simulink model "thermal_closed_loop_model"  (R2023a)
settings: Solver=VariableStepAuto  StartTime=0.0  StopTime=600  RelTol=1e-3
PostLoadFcn:
  | run('thermal_plant_h2f175_parameters.m')
  | run('thermal_plant_peripherals_parameters.m')
  | run('thermal_variants_config.m')
undefined symbols (not defined in the file or in its folder): sigbuilder_block
libraries: simulink x1, nesl_utility x1
settings Model: Creator=adrian.taveras  LastModifiedBy=stefan.notter
settings OptimizationCC: ReuseModelBlockBuffer=off

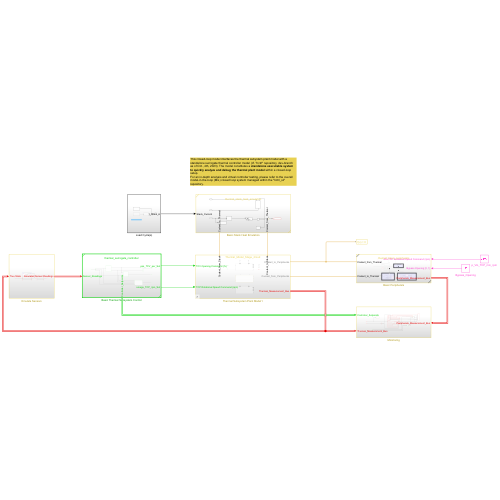
[thumbnail: Simulink's stored preview of the top-level diagram]
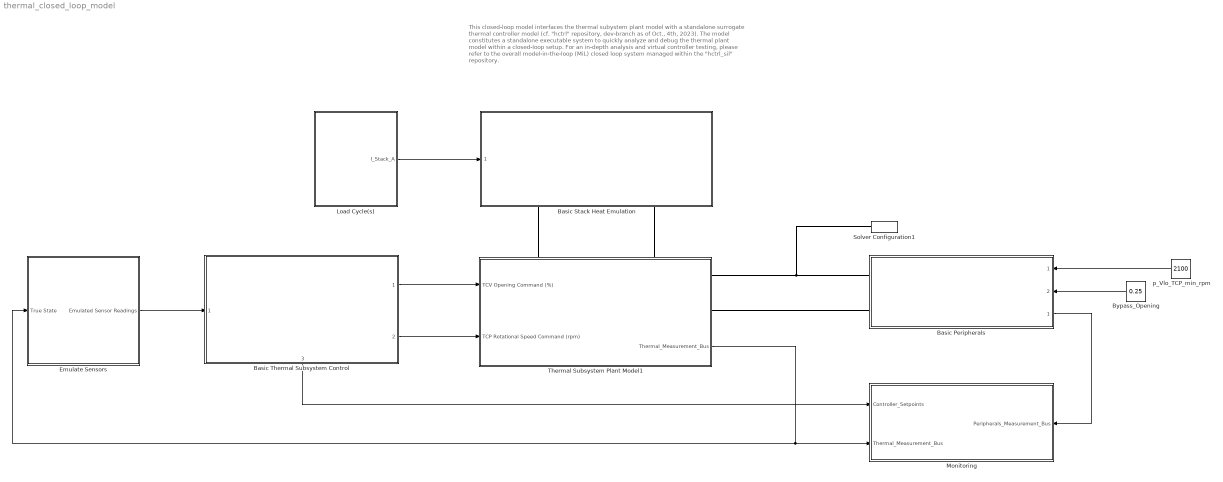
== system thermal_closed_loop_model ==
  note: This closed-loop model interfaces the thermal subystem plant model with a standalone surrogate thermal controller model (cf. "hctrl" repository, dev-branch as of Oct., 4th, 2023). The model constitutes a standalone executable system to quickly analyze and debug the thermal plant model within a closed-loop setup.
      | For an in-depth analysis and virtual controller testing, please refer to the overall model-in-the-loop (MiL) closed loop system managed within the "hctrl_sil" repository.
  Basic Peripherals : Subsystem  ReferencedSubsystem=thermal_basic_peripherals
      settings: PortSchema="{\"entries\":[{\"content\":{\"sides\":[{\"content\":{\"connectorIds\":[\"LConn1\",\"LConn2\"]},\"type\":\"ConnectorPlacement.EquallySpacedRectSide\",\"uuid\":\"3fb1bffc-06de-43a0-ba54-014616fc6cc1\"},{\"content\":{\"connectorIds\":[\"In1\",\"In2\",\"Out1\"],\"side\":\"RIGHT\"},\"type\":\"ConnectorPlacement.EquallySpacedRectSide\",\"uuid\":\"58405954-0a26-4c47-92cd-2c539f5c2dc2\"},{\"content\":{\"side\":\"TOP\"},\"type\":\"ConnectorPlacement.EquallySpacedRectSide\",\"uuid\":\"fb935e14-bdb8-42f8-ab88-5e819e25323e\"}]},\"type\":\"ConnectorPlacement.EquallySpacedConnector\",\"uuid\":\"bd863423-caf1-4028-a014-0e522635d1ca\"}],\"packageUris\":[\"http://schema.mathworks.com/mf0/Connector/R2020b\"],\"version\":\"1.0\"}"
  Basic Stack Heat Emulation : Subsystem  ReferencedSubsystem=thermal_stack_heat_emulation
      settings: PortSchema="{\"entries\":[{\"content\":{\"sides\":[{\"content\":{\"connectorIds\":[\"In1\"]},\"type\":\"ConnectorPlacement.EquallySpacedRectSide\",\"uuid\":\"3fb1bffc-06de-43a0-ba54-014616fc6cc1\"},{\"content\":{\"side\":\"RIGHT\"},\"type\":\"ConnectorPlacement.EquallySpacedRectSide\",\"uuid\":\"58405954-0a26-4c47-92cd-2c539f5c2dc2\"},{\"content\":{\"side\":\"TOP\"},\"type\":\"ConnectorPlacement.EquallySpacedRectSide\",\"uuid\":\"fb935e14-bdb8-42f8-ab88-5e819e25323e\"},{\"content\":{\"connectorIds\":[\"RConn1\",\"RConn2\"],\"side\":\"BOTTOM\"},\"type\":\"ConnectorPlacement.EquallySpacedRectSide\",\"uuid\":\"52bc4db1-df79-4132-9e52-2843fbef2d40\"}]},\"type\":\"ConnectorPlacement.EquallySpacedConnector\",\"uuid\":\"bd863423-caf1-4028-a014-0e522635d1ca\"}],\"packageUris\":[\"http://schema.mathworks.com/mf0/Connector/R2020b\"],\"version\":\"1.0\"}"
  Basic Thermal Subsystem Control : Subsystem  TreatAsAtomicUnit=on  SystemSampleTime=0.05  ReferencedSubsystem=thermal_surrogate_controller
      settings: RTWFcnNameOpts=Use subsystem name  RTWFileNameOpts=Use subsystem name  PortSchema="{\"entries\":[{\"content\":{\"sides\":[{\"content\":{\"connectorIds\":[\"In1\"]},\"type\":\"ConnectorPlacement.EquallySpacedRectSide\",\"uuid\":\"5ce399fd-075d-47cf-80d1-ee07a0b07c67\"},{\"content\":{\"connectorIds\":[\"Out1\",\"Out2\"],\"side\":\"RIGHT\"},\"type\":\"ConnectorPlacement.EquallySpacedRectSide\",\"uuid\":\"2f333d4b-83ed-4fad-b30d-41906106278f\"},{\"content\":{\"side\":\"TOP\"},\"type\":\"ConnectorPlacement.EquallySpacedRectSide\",\"uuid\":\"ce20a072-8b2c-48f8-86cd-e043d93c9dd9\"},{\"content\":{\"connectorIds\":[\"Out3\"],\"side\":\"BOTTOM\"},\"type\":\"ConnectorPlacement.EquallySpacedRectSide\",\"uuid\":\"72f45d63-3937-4d85-84da-630e4ae9e6af\"}]},\"type\":\"ConnectorPlacement.EquallySpacedConnector\",\"uuid\":\"e1990042-c5e7-41f2-bf10-f2665fc49181\"}],\"packageUris\":[\"http://schema.mathworks.com/mf0/Connector/R2020b\"],\"version\":\"1.0\"}"
  Bypass_Opening : Constant  Value=0.25
  Emulate Sensors : Subsystem
  Load Cycle(s) : Subsystem
  Monitoring : Subsystem
      settings: PortSchema="{\"entries\":[{\"content\":{\"sides\":[{\"content\":{\"connectorIds\":[\"In1\",\"In2\"]},\"type\":\"ConnectorPlacement.EquallySpacedRectSide\",\"uuid\":\"c7cb1208-b668-4b39-b890-dd3e20c5f08d\"},{\"content\":{\"connectorIds\":[\"In3\"],\"side\":\"RIGHT\"},\"type\":\"ConnectorPlacement.EquallySpacedRectSide\",\"uuid\":\"340204d2-358d-42ec-bbb6-f536bf598eab\"},{\"content\":{\"side\":\"TOP\"},\"type\":\"ConnectorPlacement.EquallySpacedRectSide\",\"uuid\":\"3db79fdc-6863-4ab5-88bc-fd1ec2b642bb\"}]},\"type\":\"ConnectorPlacement.EquallySpacedConnector\",\"uuid\":\"cd44049f-98c6-404f-bd6e-056e1be05d3b\"}],\"packageUris\":[\"http://schema.mathworks.com/mf0/Connector/R2020b\"],\"version\":\"1.0\"}"
  Solver Configuration1 : nesl_utility/Solver Configuration  PhysicalDomain=network_engine_domain  SubClassName=solver  LeftPortType=input  RightPortType=generic  Tones=[]  Harmonics=[]  SimulateNoise=off  Profile=off  UseLocalSampling=off  EnableSwitchedLinearOptims=on  FrequencyDomain=off  UseCCode=off  RelTol=0.001  AbsTol=1e-06  MinStep=1e-09  ToWorkspace=off  RevertToSquareIcSolve=off  NumHomotopyIterations=100  PhasorMode=off  PhasorModeNumHarmonics=1  ConsistencySolver=NEWTON_XTOL_AFTER_FTOL  IndexReductionMethod=DerivativeReplacement  DoDC=off  ResidualTolerance=1e-09  ConsistencyTolSource=GLOBAL  ConsistencyAbsTol=0.001  ConsistencyRelTol=0.001  ConsistencyTolFactor=0.001  UseLocalSolver=on  LocalSolverChoice=NE_BACKWARD_EULER_ADVANCER  ResolveIndetEquations=on  FunctionEvalNumThread=1  LocalSolverSampleTime=0.001  DoFixedCost=on  MaxNonlinIter=3  MaxModeIter=2  ComputeImpulses=off  ImpulseIterations=2  LinearAlgebra=auto  LinearAlgebraNumThread=0  EquationFormulation=NE_TIME_EF  DelaysMemoryBudget=1024  AutomaticFiltering=off  FilteringTimeConstant=0.001  PartitionStorageMethod=AS_NEEDED  PartitionMemoryBudget=1024  PartitionMethod=ROBUST
  Thermal Subsystem Plant Model1 : Subsystem  Variant=on
      settings: PortSchema="{\"entries\":[{\"content\":{\"sides\":[{\"content\":{\"connectorIds\":[\"In1\",\"In2\"]},\"type\":\"ConnectorPlacement.EquallySpacedRectSide\",\"uuid\":\"c406812b-8c92-4602-a172-62ad771a81a9\"},{\"content\":{\"connectorIds\":[\"RConn1\",\"RConn2\",\"Out1\"],\"side\":\"RIGHT\"},\"type\":\"ConnectorPlacement.EquallySpacedRectSide\",\"uuid\":\"78b6fff5-4256-4005-adaa-354cc2ed5b7d\"},{\"content\":{\"connectorIds\":[\"LConn1\",\"LConn2\"],\"side\":\"TOP\"},\"type\":\"ConnectorPlacement.EquallySpacedRectSide\",\"uuid\":\"1d5f4f72-4393-4f38-b9ce-f5bde53d6a3a\"}]},\"type\":\"ConnectorPlacement.EquallySpacedConnector\",\"uuid\":\"f62a8404-8485-4e42-883e-e8d18b630e2d\"}],\"packageUris\":[\"http://schema.mathworks.com/mf0/Connector/R2020b\"],\"version\":\"1.0\"}"
  p_Vlo_TCP_min_rpm : Constant  Value=2100
  wires:
  Emulate Sensors/1(Emulated Sensor Readings) -> Basic Thermal Subsystem Control/1
  p_Vlo_TCP_min_rpm/1 -> Basic Peripherals/1
  Load Cycle(s)/1(I_Stack_A) -> Basic Stack Heat Emulation/1
  Basic Peripherals/1 -> Monitoring/3(Peripherals_Measurement_Bus)
  Basic Thermal Subsystem Control/3 -> Monitoring/1(Controller_Setpoints)
  Bypass_Opening/1 -> Basic Peripherals/2
  Basic Thermal Subsystem Control/1 -> Thermal Subsystem Plant Model1/1(TCV Opening Command (%))
  Basic Thermal Subsystem Control/2 -> Thermal Subsystem Plant Model1/2(TCP Rotational Speed Command (rpm))
  Thermal Subsystem Plant Model1/1(Thermal_Measurement_Bus) -> Emulate Sensors/1(True State), Monitoring/2(Thermal_Measurement_Bus)
  connections:
  Thermal Subsystem Plant Model1/LConn2 -- Basic Stack Heat Emulation/RConn2
  Thermal Subsystem Plant Model1/LConn1 -- Basic Stack Heat Emulation/RConn1
  Thermal Subsystem Plant Model1/RConn1 -- Solver Configuration1/RConn1 -- Basic Peripherals/LConn1
  Thermal Subsystem Plant Model1/RConn2 -- Basic Peripherals/LConn2

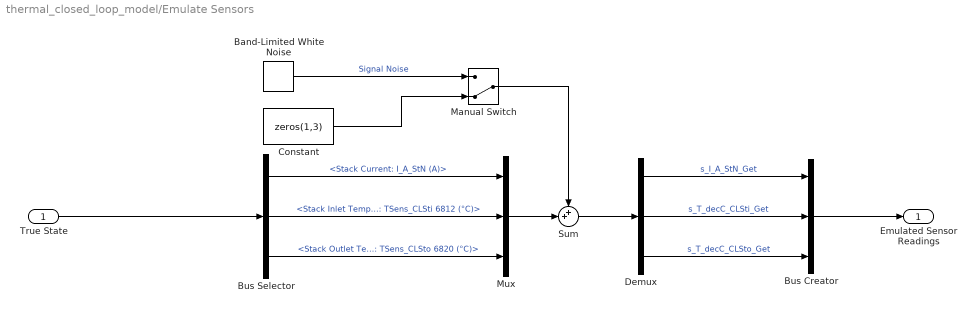
== system thermal_closed_loop_model/Emulate Sensors ==
  True State : Inport
  Band-Limited White Noise : simulink/Sources/Band-Limited White Noise  Cov=[5e-3, 5e-4, 5e-4]  Ts=0.1  seed=[23341]
  Bus Creator : BusCreator  Inputs=3
  Bus Selector : BusSelector  OutputSignals=Stack Current: I_A_StN (A),Stack Inlet Temperature: TSens_CLSti 6812 (°C),Stack Outlet Temperature: TSens_CLSto 6820 (°C)
  Constant : Constant  Value=zeros(1,3)
  Demux : Demux  Outputs=3
  Manual Switch : ManualSwitch  CurrentSetting=0
  Mux : Mux  Inputs=3
  Sum : Sum  Inputs=++|
  Emulated Sensor Readings : Outport
  wires:
  Bus Creator/1 -> Emulated Sensor Readings/1
  True State/1 -> Bus Selector/1
  Bus Selector/1 -> Mux/1  "<Stack Current: I_A_StN (A)>"
  Bus Selector/2 -> Mux/2  "<Stack Inlet Temperature: TSens_CLSti 6812 (°C)>"
  Bus Selector/3 -> Mux/3  "<Stack Outlet Temperature: TSens_CLSto 6820 (°C)>"
  Mux/1 -> Sum/2
  Sum/1 -> Demux/1
  Manual Switch/1 -> Sum/1
  Band-Limited White Noise/1 -> Manual Switch/1  "Signal Noise"
  Constant/1 -> Manual Switch/2
  Demux/1 -> Bus Creator/1  "s_I_A_StN_Get"
  Demux/3 -> Bus Creator/3  "s_T_decC_CLSto_Get"
  Demux/2 -> Bus Creator/2  "s_T_decC_CLSti_Get"

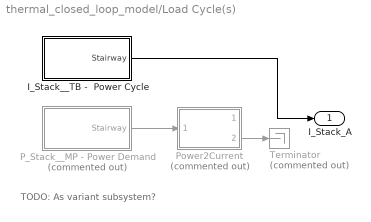
== system thermal_closed_loop_model/Load Cycle(s) ==
  note: TODO: As variant subsystem?
  I_Stack__TB -  Power Cycle : Subsystem  Tag=STV Subsys  LoadFcn=sigbuilder_block('load');  StartFcn=sigbuilder_block('start');  StopFcn=sigbuilder_block('stop');  ClipboardFcn=sigbuilder_block('clipboard');  mask(Sigbuilder block){tuvar=[0:10]}
      mask help: Simulink:masks:SigbuilderBlock_MD
      mask init:
      | if ~strcmp(get_param(bdroot(gcbh),'SimulationStatus'),'stopped') tuvar = sigbuilder_block('maskInit'); end
      settings: CopyFcn=sigbuilder_block('copy');  DeleteFcn=sigbuilder_block('delete');  ModelCloseFcn=sigbuilder_block('modelClose');  PreSaveFcn=sigbuilder_block('preSave');  PauseFcn=sigbuilder_block('pause');  ContinueFcn=sigbuilder_block('continue');  NameChangeFcn=sigbuilder_block('namechange');  OpenFcn=sigbuilder_block('open',[150.6 139.8 551.4 322.2 ]);  CloseFcn=sigbuilder_block('close');
      mask Display: plot(0, 0, 100, 100,[2, 2, 32, 32, 2], [68, 8, 8, 68, 68],[32, 2], [38, 38], [32, 19, 2],[53, 60, 44], [32, 17, 17, 2],[16, 16, 31, 31]);txt = getActiveGroup(gcbh);text(2, 100, txt,'verticalAlignment', 'top');
  P_Stack__MP - Power Demand : Subsystem  Tag=STV Subsys  Commented=on  LoadFcn=sigbuilder_block('load');  StartFcn=sigbuilder_block('start');  StopFcn=sigbuilder_block('stop');  ClipboardFcn=sigbuilder_block('clipboard');  mask(Sigbuilder block){tuvar=[0:10]}
      mask help: Simulink:masks:SigbuilderBlock_MD
      mask init:
      | if ~strcmp(get_param(bdroot(gcbh),'SimulationStatus'),'stopped') tuvar = sigbuilder_block('maskInit'); end
      settings: CopyFcn=sigbuilder_block('copy');  DeleteFcn=sigbuilder_block('delete');  ModelCloseFcn=sigbuilder_block('modelClose');  PreSaveFcn=sigbuilder_block('preSave');  PauseFcn=sigbuilder_block('pause');  ContinueFcn=sigbuilder_block('continue');  NameChangeFcn=sigbuilder_block('namechange');  OpenFcn=sigbuilder_block('open',[5.4 5.4 1141.2 580.8 ]);  CloseFcn=sigbuilder_block('close');
      mask Display: plot(0, 0, 100, 100,[2, 2, 32, 32, 2], [68, 8, 8, 68, 68],[32, 2], [38, 38], [32, 19, 2],[53, 60, 44], [32, 17, 17, 2],[16, 16, 31, 31]);txt = getActiveGroup(gcbh);text(2, 100, txt,'verticalAlignment', 'top');
  Power2Current : Subsystem  Commented=on
  Terminator : Terminator  Commented=on
  I_Stack_A : Outport
  wires:
  P_Stack__MP - Power Demand/1(Stairway) -> Power2Current/1(P_Stack)
  Power2Current/2(V_Stack) -> Terminator/1
  I_Stack__TB -  Power Cycle/1(Stairway) -> I_Stack_A/1

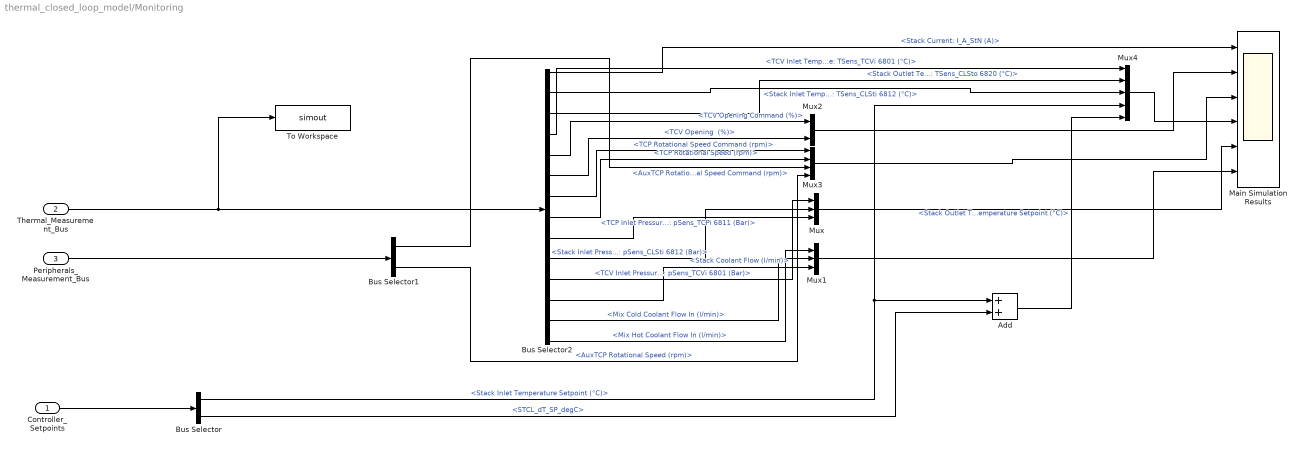
== system thermal_closed_loop_model/Monitoring ==
  Controller_Setpoints : Inport
  Thermal_Measurement_Bus : Inport  Port=2
  Peripherals_Measurement_Bus : Inport  Port=3
  Add : Sum
  Bus Selector : BusSelector  OutputSignals=Stack Inlet Temperature Setpoint (°C),STCL_dT_SP_degC
  Bus Selector1 : BusSelector  OutputSignals=AuxTCP Rotational Speed Command (rpm),AuxTCP Rotational Speed (rpm)
  Bus Selector2 : BusSelector  OutputSignals="Stack Current: I_A_StN (A),Stack Inlet Temperature: TSens_CLSti 6812 (°C),Stack Outlet Temperature: TSens_CLSto 6820 (°C),TCV Inlet Temperature: TSens_TCVi 6801 (°C),TCV Opening Command (%),TCV Opening  (%),TCP Rotational Speed Command (rpm),TCP Rotational Speed (rpm),TCP Inlet Pressure: pSens_TCPi 6811 (Bar),Stack Inlet Pressure: pSens_CLSti 6812 (Bar),TCV Inlet Pressure: pSens_TCVi 6801 (Bar),Stack Coolant Flow (l/min),Mix Cold Coolant Flow In (l/min),Mix Hot Coolant Flow In (l/min)"
  Main Simulation Results : Scope  NumInputPorts=6
  Mux : Mux  Inputs=3
  Mux1 : Mux  Inputs=3
  Mux2 : Mux  Inputs=2
  Mux3 : Mux
  Mux4 : Mux  Inputs=5
  To Workspace : ToWorkspace  VariableName=simout  SaveFormat=Timeseries  SampleTime=-1
  wires:
  Mux4/1 -> Main Simulation Results/4
  Bus Selector2/9 -> Mux/3  "<TCP Inlet Pressure: pSens_TCPi 6811 (Bar)>"
  Mux3/1 -> Main Simulation Results/3
  Bus Selector2/7 -> Mux3/1  "<TCP Rotational Speed Command (rpm)>"
  Bus Selector2/3 -> Mux4/2  "<Stack Outlet Temperature: TSens_CLSto 6820 (°C)>"
  Mux2/1 -> Main Simulation Results/2
  Thermal_Measurement_Bus/1 -> To Workspace/1, Bus Selector2/1
  Bus Selector2/2 -> Mux4/3  "<Stack Inlet Temperature: TSens_CLSti 6812 (°C)>"
  Bus Selector2/6 -> Mux2/2  "<TCV Opening  (%)>"
  Mux/1 -> Main Simulation Results/5
  Bus Selector2/13 -> Mux1/2  "<Mix Cold Coolant Flow In (l/min)>"
  Bus Selector2/11 -> Mux/1  "<TCV Inlet Pressure: pSens_TCVi 6801 (Bar)>"
  Bus Selector2/12 -> Mux1/3  "<Stack Coolant Flow (l/min)>"
  Mux1/1 -> Main Simulation Results/6
  Bus Selector2/8 -> Mux3/2  "<TCP Rotational Speed (rpm)>"
  Bus Selector2/5 -> Mux2/1  "<TCV Opening Command (%)>"
  Bus Selector2/14 -> Mux1/1  "<Mix Hot Coolant Flow In (l/min)>"
  Bus Selector2/10 -> Mux/2  "<Stack Inlet Pressure: pSens_CLSti 6812 (Bar)>"
  Bus Selector2/4 -> Mux4/1  "<TCV Inlet Temperature: TSens_TCVi 6801 (°C)>"
  Bus Selector2/1 -> Main Simulation Results/1  "<Stack Current: I_A_StN (A)>"
  Peripherals_Measurement_Bus/1 -> Bus Selector1/1
  Bus Selector1/1 -> Mux3/3  "<AuxTCP Rotational Speed Command (rpm)>"
  Bus Selector1/2 -> Mux3/4  "<AuxTCP Rotational Speed (rpm)>"
  Bus Selector/2 -> Add/2  "<STCL_dT_SP_degC>"
  Add/1 -> Mux4/5  "<Stack Outlet Temperature Setpoint (°C)>"
  Controller_Setpoints/1 -> Bus Selector/1
  Bus Selector/1 -> Add/1, Mux4/4  "<Stack Inlet Temperature Setpoint (°C)>"

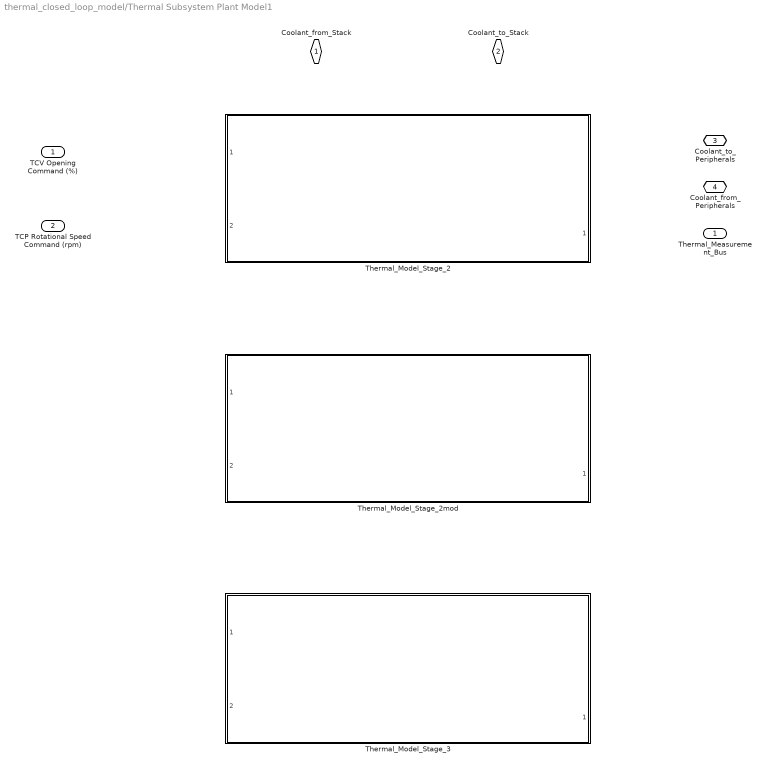
== system thermal_closed_loop_model/Thermal Subsystem Plant Model1 ==
  TCV Opening Command (%) : Inport
  TCP Rotational Speed Command (rpm) : Inport  Port=2
  Thermal_Model_Stage_2 : Subsystem  VariantControl=THERMALMODEL_VARIANT_STAGE_TWO  ReferencedSubsystem=thermal_model_stage_2
      settings: PortSchema="{\"entries\":[{\"content\":{\"sides\":[{\"content\":{\"connectorIds\":[\"In1\",\"In2\"]},\"type\":\"ConnectorPlacement.EquallySpacedRectSide\",\"uuid\":\"beafa6ad-25d9-43ec-83ed-6cc27c4ae524\"},{\"content\":{\"connectorIds\":[\"RConn1\",\"RConn2\",\"Out1\"],\"side\":\"RIGHT\"},\"type\":\"ConnectorPlacement.EquallySpacedRectSide\",\"uuid\":\"0e4b084f-16c4-4479-9add-ada13fc3130c\"},{\"content\":{\"connectorIds\":[\"LConn2\",\"LConn1\"],\"side\":\"TOP\"},\"type\":\"ConnectorPlacement.EquallySpacedRectSide\",\"uuid\":\"1a5fc455-48ce-4ccf-a3dc-1364efaff46d\"}]},\"type\":\"ConnectorPlacement.EquallySpacedConnector\",\"uuid\":\"dcdc6280-b7d6-42a7-acf0-0a1a3b6a3e13\"}],\"packageUris\":[\"http://schema.mathworks.com/mf0/Connector/R2020b\"],\"version\":\"1.0\"}"
  Thermal_Model_Stage_2mod : Subsystem  VariantControl=THERMALMODEL_VARIANT_STAGE_TWO_MOD  ReferencedSubsystem=thermal_model_stage_2_mod
      settings: PortSchema="{\"entries\":[{\"content\":{\"sides\":[{\"content\":{\"connectorIds\":[\"In1\",\"In2\"]},\"type\":\"ConnectorPlacement.EquallySpacedRectSide\",\"uuid\":\"beafa6ad-25d9-43ec-83ed-6cc27c4ae524\"},{\"content\":{\"connectorIds\":[\"RConn1\",\"RConn2\",\"Out1\"],\"side\":\"RIGHT\"},\"type\":\"ConnectorPlacement.EquallySpacedRectSide\",\"uuid\":\"0e4b084f-16c4-4479-9add-ada13fc3130c\"},{\"content\":{\"connectorIds\":[\"LConn2\",\"LConn1\"],\"side\":\"TOP\"},\"type\":\"ConnectorPlacement.EquallySpacedRectSide\",\"uuid\":\"1a5fc455-48ce-4ccf-a3dc-1364efaff46d\"}]},\"type\":\"ConnectorPlacement.EquallySpacedConnector\",\"uuid\":\"dcdc6280-b7d6-42a7-acf0-0a1a3b6a3e13\"}],\"packageUris\":[\"http://schema.mathworks.com/mf0/Connector/R2020b\"],\"version\":\"1.0\"}"
  Thermal_Model_Stage_3 : Subsystem  VariantControl=THERMALMODEL_VARIANT_STAGE_THREE  ReferencedSubsystem=thermal_model_stage_3
      settings: PortSchema="{\"entries\":[{\"content\":{\"sides\":[{\"content\":{\"connectorIds\":[\"In1\",\"In2\"]},\"type\":\"ConnectorPlacement.EquallySpacedRectSide\",\"uuid\":\"beafa6ad-25d9-43ec-83ed-6cc27c4ae524\"},{\"content\":{\"connectorIds\":[\"RConn1\",\"RConn2\",\"Out1\"],\"side\":\"RIGHT\"},\"type\":\"ConnectorPlacement.EquallySpacedRectSide\",\"uuid\":\"0e4b084f-16c4-4479-9add-ada13fc3130c\"},{\"content\":{\"connectorIds\":[\"LConn2\",\"LConn1\"],\"side\":\"TOP\"},\"type\":\"ConnectorPlacement.EquallySpacedRectSide\",\"uuid\":\"1a5fc455-48ce-4ccf-a3dc-1364efaff46d\"}]},\"type\":\"ConnectorPlacement.EquallySpacedConnector\",\"uuid\":\"dcdc6280-b7d6-42a7-acf0-0a1a3b6a3e13\"}],\"packageUris\":[\"http://schema.mathworks.com/mf0/Connector/R2020b\"],\"version\":\"1.0\"}"
  Coolant_from_Stack : PMIOPort  Side=Left
  Coolant_to_Stack : PMIOPort  Port=2  Side=Left
  Coolant_to_Peripherals : PMIOPort  Port=3  Side=Right
  Coolant_from_Peripherals : PMIOPort  Port=4  Side=Right
  Thermal_Measurement_Bus : Outport

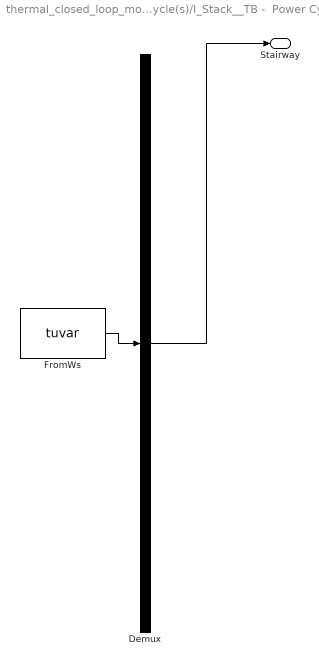
== system thermal_closed_loop_model/Load Cycle(s)/I_Stack__TB -  Power Cycle ==
  Demux : Demux  Tag=STV Demux  Outputs=1
      settings: DisplayOption=none
  FromWs : FromWorkspace  Tag=STV FromWs  VariableName=tuvar
      SigBuilderData=|
      | common.afterFinalStr = 'Extrapolate'
      | common.sampleTime = 0
      | dataSet.timeRange = [0 600]
      | dataSet.name = 'Group 1'
      | sbobj.Groups.Name = 'Group 1'
      | sbobj.Groups.Signals.Name = 'Stairway'
      | sbobj.Groups.Signals.XData = [0 180 190 250 260 320 330 390 400 460 470 530 540 600]
      | sbobj.Groups.Signals.YData = [100 100 200 200 300 300 400 400 300 300 200 200 100 100]
      | sbobj.Groups.TimeRange = [0 600]
  Stairway : Outport  Tag=STV Outport
  wires:
  Demux/1 -> Stairway/1
  FromWs/1 -> Demux/1

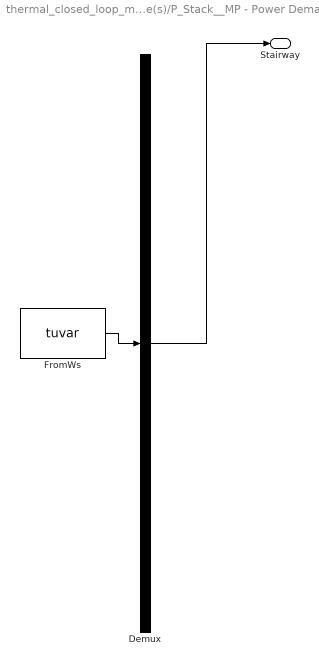
== system thermal_closed_loop_model/Load Cycle(s)/P_Stack__MP - Power Demand ==
  Demux : Demux  Tag=STV Demux  Outputs=1
      settings: DisplayOption=none
  FromWs : FromWorkspace  Tag=STV FromWs  VariableName=tuvar
      SigBuilderData=|
      | common.afterFinalStr = 'Extrapolate'
      | common.sampleTime = 0
      | dataSet.timeRange = [0 22226]
      | dataSet.name = 'Group 1'
      | sbobj.Groups.Name = 'Group 1'
      | sbobj.Groups.Signals.Name = 'Stairway'
      | sbobj.Groups.Signals.XData = [0 1 1.1 1.2 1.3 60 120 5000 5000 21146 21826 22226]
      | sbobj.Groups.Signals.YData = [0 0 0 0 1 1 100 100 85 85 25 1]
      | sbobj.Groups.TimeRange = [0 22226]
  Stairway : Outport  Tag=STV Outport
  wires:
  FromWs/1 -> Demux/1
  Demux/1 -> Stairway/1

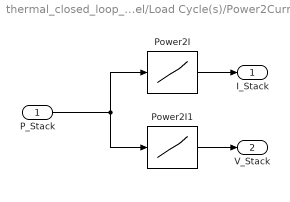
== system thermal_closed_loop_model/Load Cycle(s)/Power2Current ==
  P_Stack : Inport
  Power2I : Lookup_n-D  NumberOfTableDimensions=1  BreakpointsForDimension1=[0;8.5;17;26;34;42;50;58.3;66.66;85;100]  Table=[0;50;100;150;200;250;300;350;400;510;600]  InternalRulePriority=Speed  RndMeth=Simplest
  Power2I1 : Lookup_n-D  NumberOfTableDimensions=1  BreakpointsForDimension1=[0;8.5;17;26;34;42;50;58.3;66.66;85;100]  Table=[370;350;330;310;290;270;250;226;210;186;166.66]  InternalRulePriority=Speed  RndMeth=Simplest
  I_Stack : Outport
  V_Stack : Outport  Port=2
  wires:
  P_Stack/1 -> Power2I1/1, Power2I/1
  Power2I/1 -> I_Stack/1
  Power2I1/1 -> V_Stack/1
